simulink model "Gyro_Outage_Unit_Test"  (R2018b)
settings: Solver=VariableStepAuto  StartTime=0.0  StopTime=5600  FixedStep=fswParams.sample_time_s  RelTol=1e-8  AbsTol=1e-8
undefined symbols (not defined in the file or in its folder): B_eci_unit, Conversion_lib, DiscIntNeverNeededParam, e2sun_eci_unit, ECLIPSE, env_acc_mps2, Environment_lib, fswParams, gyro_body_radps, gyro_meas_valid, mag_body_T, mag_meas_valid, MEKF_Conversion_lib, MEKF_lib, photodiodes_A, q_body, r_eci_km, satelliteDynamics_lib, sc2sun_eci_unit, Sensors_Lib, simParams, solar_panel_power_W, sun_sensor_lib, sunsensor_2body_lib, sunsensor_body_deg, sunsensor_body_rad, sunsensor_valid, Triad, Triad_lib, v_eci_km, w_body_radps
libraries: aerolibutil x11, vrlib x10, sharedutil x8, simulink x5, dspmathops x4, sharedtransform x3, magnetometer_lib x3, gyroscope_lib x2, gravityGrad_Lib x1, atmoDrag_lib x1, magField_lib x1, solarPressure_lib x1
(part 2 of 3)

== system Gyro_Outage_Unit_Test/MEKF_lib1/Time Propagation (q,P) ==
  qe_plus : Inport
  P_chol_plus : Inport  Port=2
  Updated bias : Inport  Port=3
  omega_meas : Inport  Port=4
  Constant : Constant  Value=fswParams.estimation.dt
  Constant13 : Constant  Value=fswParams.estimation.Qchol  VectorParams1D=off
  Cross_Product_matrix : Subsystem
  Cross_product_matrix : Subsystem
  MATLAB Function : MATLAB Function  TreatAsAtomicUnit=on
  MATLAB Function10 : MATLAB Function  TreatAsAtomicUnit=on
  Matrix Multiply : Product  Multiplication=Matrix(*)
  Product : Product  Multiplication=Matrix(*)
  Psi : Subsystem
  Quaternion Normalize : sharedutil/Quaternion Normalize  aMode=aMode
      settings: SourceProductName=Aerospace Blockset  SourceProductBaseCode=AE
  Rate Transition : RateTransition  InitialCondition=fswParams.estimation.ic.Qchol_rt  OutPortSampleTime=fswParams.sample_time_s
  Sqrt : Sqrt  SaturateOnIntegerOverflow=on
  Subsystem : Subsystem
  Sum : Sum  Inputs=+-
  Transpose : Math  Operator=transpose  SaturateOnIntegerOverflow=on
  q_k_plus1 : Outport
  P_chol_plus_1 : Outport  Port=2
  Bias_Update : Outport  Port=3
  omega_est : Outport  Port=4
  wires:
  Quaternion Normalize/1 -> q_k_plus1/1
  omega_meas/1 -> Sum/1
  Product/1 -> Quaternion Normalize/1
  [del_t] -> MATLAB Function10/3(dt)
  qe_plus/1 -> Product/2
  [del_t] -> Psi/1(del_t)
  Sum/1 -> Cross_Product_matrix/1(omega_est), Matrix Multiply/2, omega_est/1, Psi/2(omega_vec), Transpose/1  "omega_estimate"
  Constant/1 -> [del_t]
  Matrix Multiply/1 -> Sqrt/1
  Transpose/1 -> Matrix Multiply/1
  Updated bias/1 -> Bias_Update/1, Sum/2
  Sqrt/1 -> MATLAB Function10/1(om_mag), Psi/3(omega_mag), Subsystem/4(omega_magnitude)  "omega_magnitude"
  Cross_Product_matrix/1(omega_x) -> MATLAB Function10/2(omega_x)
  [del_t] -> Subsystem/1(del_t)
  Psi/1(Psi1) -> Subsystem/3(Psi_vector), Cross_product_matrix/1(Psi_vec)  "Psi Vector"
  Cross_product_matrix/1(Psi_x) -> Subsystem/2(Psi_cross)
  Subsystem/1(OMEGA) -> Product/1
  Constant13/1 -> Rate Transition/1
  MATLAB Function10/1(Phi) -> MATLAB Function/2(Phi_discrete)  "State Transition Matrix"
  P_chol_plus/1 -> MATLAB Function/1("P_sq ")
  MATLAB Function/1(P_sq) -> P_chol_plus_1/1
  Rate Transition/1 -> MATLAB Function/3(Q_sq)

== system Gyro_Outage_Unit_Test/MEKF_lib1/Triad ==
  sc2sun_eci_unit : Inport
  B_eci_unit : Inport  Port=2
  sun_meas_rad_body : Inport  Port=3
  mag_meas_body_T : Inport  Port=4
  sunsensor_valid : Inport  Port=5
  magsensor_valid : Inport  Port=6
  Action Port : ActionPort
  Angle_between_vectors : Subsystem
  Bypass Triad : Subsystem  TreatAsAtomicUnit=on
  If : If  IfExpression=u1
  Logical Operator : Logic  Inputs=3  AllPortsSameDT=off  OutDataTypeStr=boolean
  Merge : Merge
  Quaternion Normalize : sharedutil/Quaternion Normalize  aMode=aMode
      settings: SourceProductName=Aerospace Blockset  SourceProductBaseCode=AE
  Triad_alg : Subsystem  TreatAsAtomicUnit=on
  Unit Delay : UnitDelay  InitialCondition=fswParams.estimation.ic.quat_est_init  SampleTime=fswParams.sample_time_s
  q_triad : Outport
  wires:
  Merge/1 -> Quaternion Normalize/1, [quat_old]
  Quaternion Normalize/1 -> q_triad/1
  If/1 -> Triad_alg/Action
  If/2 -> Bypass Triad/Action
  Triad_alg/1(quat_out 2) -> Merge/1
  Bypass Triad/1(quat_new) -> Merge/2
  Logical Operator/1 -> If/1
  sunsensor_valid/1 -> Logical Operator/1
  magsensor_valid/1 -> Logical Operator/2
  B_eci_unit/1 -> Triad_alg/3("mag_inertial ")
  [quat_old] -> Unit Delay/1
  Unit Delay/1 -> Bypass Triad/1(quat_old)
  sc2sun_eci_unit/1 -> Triad_alg/4(sun_inertial)
  sun_meas_rad_body/1 -> [sun_bod], Angle_between_vectors/1(sun_meas_rad_body)
  mag_meas_body_T/1 -> Angle_between_vectors/2(mag_meas_T_body), [meas_bod]
  Angle_between_vectors/1(Parallel_Protection) -> Logical Operator/3
  [sun_bod] -> Triad_alg/1(sun_body)
  [meas_bod] -> Triad_alg/2(mag_body)

== system Gyro_Outage_Unit_Test/MEKF_lib2/Angle_between_vectors ==
  sun_meas_rad_body : Inport
  mag_meas_T_body : Inport  Port=2
  Acos1 : Trigonometry  Commented=through  Operator=acos
  Divide : Product  Inputs=*/
  Dot Product : DotProduct  InputSameDT=on  OutDataTypeStr=Inherit: Inherit via internal rule
  Dot Product1 : DotProduct  InputSameDT=on  OutDataTypeStr=Inherit: Inherit via internal rule
  Dot Product2 : DotProduct  InputSameDT=on  OutDataTypeStr=Inherit: Inherit via internal rule
  Gain1 : Gain  Commented=through  Gain=180/pi
  MATLAB Function : MATLAB Function  TreatAsAtomicUnit=on
  Multiply : Product
  Multiply1 : Product
  Scope : Scope
  Sign : Signum
  Sqrt : Sqrt  SaturateOnIntegerOverflow=on
  Sqrt1 : Sqrt  SaturateOnIntegerOverflow=on
  Out1 : Outport
  wires:
  Dot Product1/1 -> Sqrt/1
  mag_meas_T_body/1 -> Dot Product2/2, Dot Product2/1, Dot Product/2
  sun_meas_rad_body/1 -> Dot Product1/1, Dot Product1/2, Dot Product/1
  Sqrt1/1 -> Multiply/2
  Sqrt/1 -> Multiply/1
  Dot Product/1 -> Divide/1
  Dot Product2/1 -> Sqrt1/1
  Multiply/1 -> Divide/2
  Acos1/1 -> Gain1/1
  Divide/1 -> Multiply1/1, Sign/1
  Multiply1/1 -> MATLAB Function/1(u)
  Sign/1 -> Multiply1/2
  MATLAB Function/1(y) -> Scope/1, Out1/1

== system Gyro_Outage_Unit_Test/MEKF_lib2/If Action Subsystem1 ==
  P (-) : Inport
  Bias (-) : Inport  Port=2
  q (-) : Inport  Port=3
  Action Port : ActionPort  ActionType=else
  q (+) : Outport
  P (+) : Outport  Port=2
  Bias (+) : Outport  Port=3
  wires:
  P (-)/1 -> P (+)/1
  Bias (-)/1 -> Bias (+)/1
  q (-)/1 -> q (+)/1

== system Gyro_Outage_Unit_Test/MEKF_lib2/If Action Subsystem2 ==
  In1 : Inport
  Action Port : ActionPort  ActionType=else
  Out1 : Outport
  wires:
  In1/1 -> Out1/1

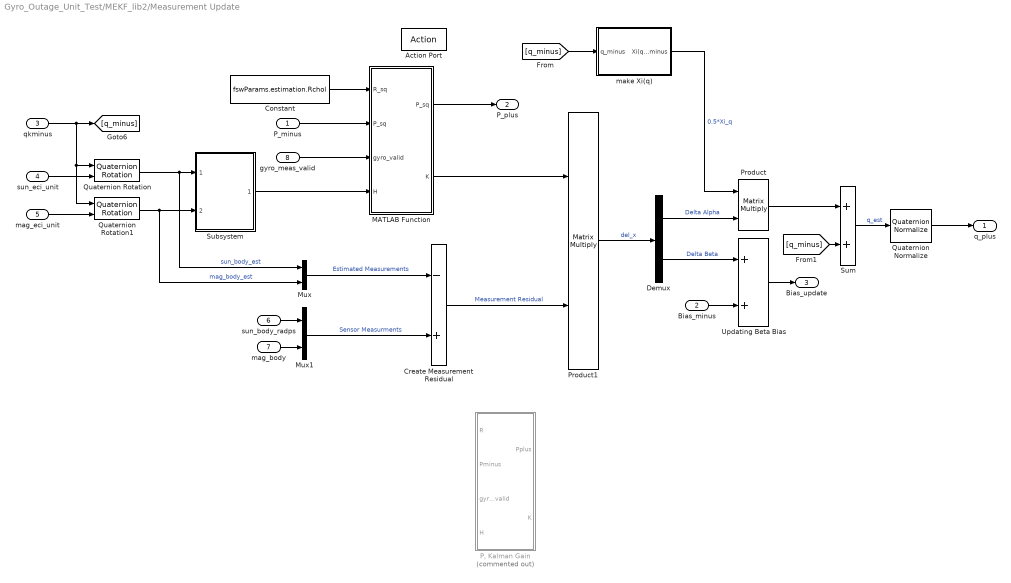
== system Gyro_Outage_Unit_Test/MEKF_lib2/Measurement Update ==
  P_minus : Inport
  Bias_minus : Inport  Port=2
  qkminus : Inport  Port=3
  sun_eci_unit : Inport  Port=4
  mag_eci_unit : Inport  Port=5
  sun_body_radps : Inport  Port=6
  mag_body : Inport  Port=7
  gyro_meas_valid : Inport  Port=8
  Action Port : ActionPort  ActionType=then
  Constant : Constant  Value=fswParams.estimation.Rchol  VectorParams1D=off
  Create Measurement Residual : Sum  Inputs=-+
  Demux : Demux  Outputs=2
  MATLAB Function : MATLAB Function  TreatAsAtomicUnit=on
  Mux : Mux  Inputs=2
  Mux1 : Mux  Inputs=2
  "P, Kalman Gain" : MATLAB Function  Commented=on  TreatAsAtomicUnit=on
  Product : Product  Inputs=**  Multiplication=Matrix(*)
  Product1 : Product  Multiplication=Matrix(*)
  Quaternion Normalize : sharedutil/Quaternion Normalize  aMode=aMode
      settings: SourceProductName=Aerospace Blockset  SourceProductBaseCode=AE
  Quaternion Rotation : aerolibutil/Quaternion Rotation
  Quaternion Rotation1 : aerolibutil/Quaternion Rotation
  Subsystem : Subsystem
  Sum : Sum
  "Updating Beta Bias " : Sum
  make Xi(q) : Subsystem
  q_plus : Outport
  P_plus : Outport  Port=2
  Bias_update : Outport  Port=3
  wires:
  MATLAB Function/2(K) -> Product1/1
  MATLAB Function/1(P_sq) -> P_plus/1
  Subsystem/1(H_matrix) -> MATLAB Function/4(H)
  gyro_meas_valid/1 -> MATLAB Function/3(gyro_valid)
  P_minus/1 -> MATLAB Function/2("P_sq ")
  Constant/1 -> MATLAB Function/1(R_sq)
  [q_minus] -> make Xi(q)/1(q_minus)
  qkminus/1 -> [q_minus], Quaternion Rotation/1, Quaternion Rotation1/1
  Quaternion Rotation/1 -> Mux/1, Subsystem/1(sun_body_hat)  "sun_body_est"
  Quaternion Rotation1/1 -> Mux/2, Subsystem/2(mag_body_hat)  "mag_body_est"
  mag_eci_unit/1 -> Quaternion Rotation1/2
  sun_eci_unit/1 -> Quaternion Rotation/2
  "Updating Beta Bias "/1 -> Bias_update/1
  sun_body_radps/1 -> Mux1/1
  mag_body/1 -> Mux1/2
  Create Measurement Residual/1 -> Product1/2  "Measurement Residual"
  make Xi(q)/1(Xi(q)_minus) -> Product/1  "0.5*Xi_q"
  Demux/1 -> Product/2  "Delta Alpha"
  Product1/1 -> Demux/1  "del_x"
  Product/1 -> Sum/1
  Sum/1 -> Quaternion Normalize/1  "q_est"
  Bias_minus/1 -> "Updating Beta Bias "/2
  Mux/1 -> Create Measurement Residual/1  "Estimated Measurements"
  Demux/2 -> "Updating Beta Bias "/1  "Delta Beta"
  Mux1/1 -> Create Measurement Residual/2  "Sensor Measurments"
  [q_minus] -> Sum/2
  Quaternion Normalize/1 -> q_plus/1

== system Gyro_Outage_Unit_Test/MEKF_lib2/Three_sigma ==
  P_plus : Inport
  Abs : Abs
  Demux : Demux  Outputs=2
  Extract Diagonal : S-Function  AncestorBlock=dspmtrx3/Extract Diagonal  FunctionName=sdspdiag2  Parameters=mode  SFunctionDeploymentMode=off  EnableBusSupport=off  mask(Extract Diagonal){}
      mask help: Extract the main diagonal of a full matrix.
      mask init:
      | mode = 2;
      | x = [.58 .87 NaN 0.12 0.45 0.45 0.12 0.12 NaN 0.525 0.525 0.475 0.475 0.525 0.525 0.565 0.525 ];
      | y = [ 0.8 0.2 NaN 0.2 0.2 0.8 0.8 0.2 NaN 0.435 0.475 0.475 0.525 0.525 0.565 0.5 0.435 ];
      mask Help: eval('blocksethelp');
      mask Display:
      | plot(x,y);
      | port_label('input',1,'A');
      | port_label('output',1,'D');
  Multiply : Gain  Gain=3*180/pi
  Terminator : Terminator
  3Sigma_deg : Outport
  wires:
  Demux/2 -> Terminator/1
  Demux/1 -> Abs/1
  Extract Diagonal/1 -> Demux/1
  Abs/1 -> Multiply/1
  P_plus/1 -> Extract Diagonal/1
  Multiply/1 -> 3Sigma_deg/1

== system Gyro_Outage_Unit_Test/MEKF_lib2/Time Propagation (q,P) ==
  qe_plus : Inport
  P_plus : Inport  Port=2
  Updated bias : Inport  Port=3
  omega_meas : Inport  Port=4
  Constant : Constant  Value=fswParams.estimation.dt
  Constant13 : Constant  Value=fswParams.estimation.Qchol  VectorParams1D=off
  Cross_Product_matrix : Subsystem
  Cross_product_matrix : Subsystem
  MATLAB Function : MATLAB Function  TreatAsAtomicUnit=on
  MATLAB Function1 : MATLAB Function  Commented=on  TreatAsAtomicUnit=on
  MATLAB Function10 : MATLAB Function  TreatAsAtomicUnit=on
  Matrix Multiply : Product  Multiplication=Matrix(*)
  Product : Product  Multiplication=Matrix(*)
  Psi : Subsystem
  Quaternion Normalize : sharedutil/Quaternion Normalize  aMode=aMode
      settings: SourceProductName=Aerospace Blockset  SourceProductBaseCode=AE
  Sqrt : Sqrt  SaturateOnIntegerOverflow=on
  Subsystem : Subsystem
  Sum : Sum  Inputs=+-
  Transpose : Math  Operator=transpose  SaturateOnIntegerOverflow=on
  P_k_plus1 : Outport
  q_k_plus1 : Outport  Port=2
  omega_est : Outport  Port=3
  Bias_Update : Outport  Port=4
  wires:
  MATLAB Function/1(P_sq) -> P_k_plus1/1
  P_plus/1 -> MATLAB Function/1("P_sq ")
  MATLAB Function10/1(Phi) -> MATLAB Function/2(Phi_discrete)  "State Transition Matrix"
  Constant13/1 -> MATLAB Function/3(Q_sq)
  Subsystem/1(OMEGA) -> Product/1
  Cross_product_matrix/1(Psi_x) -> Subsystem/2(Psi_cross)
  Psi/1(Psi1) -> Cross_product_matrix/1(Psi_vec), Subsystem/3(Psi_vector)  "Psi Vector"
  [del_t] -> Subsystem/1(del_t)
  Cross_Product_matrix/1(omega_x) -> MATLAB Function10/2(omega_x)
  Sqrt/1 -> Subsystem/4(omega_magnitude), Psi/3(omega_mag), MATLAB Function10/1(om_mag)  "omega_magnitude"
  Updated bias/1 -> Sum/2, Bias_Update/1
  Transpose/1 -> Matrix Multiply/1
  Matrix Multiply/1 -> Sqrt/1
  Constant/1 -> [del_t]
  Sum/1 -> Transpose/1, Psi/2(omega_vec), omega_est/1, Matrix Multiply/2, Cross_Product_matrix/1(omega_est)  "omega_estimate"
  [del_t] -> Psi/1(del_t)
  qe_plus/1 -> Product/2
  [del_t] -> MATLAB Function10/3(dt)
  Product/1 -> Quaternion Normalize/1
  omega_meas/1 -> Sum/1
  Quaternion Normalize/1 -> q_k_plus1/1

== system Gyro_Outage_Unit_Test/MEKF_lib2/Triad ==
  sc2sun_eci_unit : Inport
  B_eci_unit : Inport  Port=2
  sun_body_rad : Inport  Port=3
  mag_body_T : Inport  Port=4
  sunsensor_valid : Inport  Port=5
  magsensor_valid : Inport  Port=6
  Parallel_meas_check : Inport  Port=7
  Action Port : ActionPort  ActionType=then
  Bypass Triad : Subsystem  TreatAsAtomicUnit=on
  If : If  IfExpression=u1
  Logical Operator : Logic  Inputs=3  AllPortsSameDT=off  OutDataTypeStr=boolean
  Merge : Merge
  Quaternion Normalize : sharedutil/Quaternion Normalize  aMode=aMode
      settings: SourceProductName=Aerospace Blockset  SourceProductBaseCode=AE
  Triad_alg : Subsystem  TreatAsAtomicUnit=on
  Unit Delay : UnitDelay  InitialCondition=[0;0.707106781186547;0.707106781186547;0]  SampleTime=fswParams.sample_time_s
  q_triad : Outport
  wires:
  sc2sun_eci_unit/1 -> Triad_alg/4(sun_inertial)
  Unit Delay/1 -> Bypass Triad/1(quat_old)
  [quat_old] -> Unit Delay/1
  B_eci_unit/1 -> Triad_alg/3("mag_inertial ")
  sun_body_rad/1 -> Triad_alg/1(sun_body)
  mag_body_T/1 -> Triad_alg/2(mag_body)
  magsensor_valid/1 -> Logical Operator/2
  sunsensor_valid/1 -> Logical Operator/1
  Logical Operator/1 -> If/1
  Bypass Triad/1(quat_new) -> Merge/2
  Triad_alg/1(quat_out 2) -> Merge/1
  If/2 -> Bypass Triad/Action
  If/1 -> Triad_alg/Action
  Quaternion Normalize/1 -> q_triad/1
  Merge/1 -> [quat_old], Quaternion Normalize/1
  Parallel_meas_check/1 -> Logical Operator/3

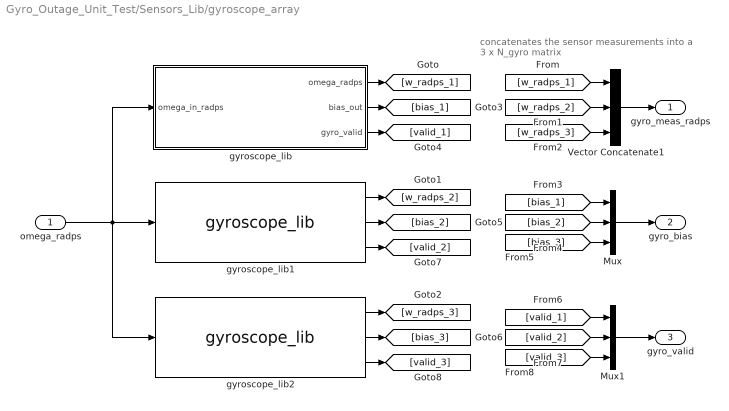
== system Gyro_Outage_Unit_Test/Sensors_Lib/gyroscope_array ==
  note: concatenates the sensor measurements
      | into a 3 x N_gyro matrix
  omega_radps : Inport
  Mux : Mux  Inputs=3
  Mux1 : Mux  Inputs=3
  Vector Concatenate1 : Concatenate  NumInputs=3  Mode=Multidimensional array  ConcatenateDimension=2
  gyroscope_lib : Subsystem  AncestorBlock=gyroscope_lib/gyroscope_lib  mask{id_s=1}
      mask prompts: id_s "Choose the sensor ID"
      mask TypeOptions id_s: 1 | 2 | 3
      mask DialogControl DescTextVar Prompt: SOCi gyroscope model. The spacecraft has three Bosch BMI055 gyroscopes.
  gyroscope_lib1 : gyroscope_lib/gyroscope_lib  id_s=2
  gyroscope_lib2 : gyroscope_lib/gyroscope_lib  id_s=3
  gyro_meas_radps : Outport
  gyro_bias : Outport  Port=2
  gyro_valid : Outport  Port=3
  wires:
  [valid_3] -> Mux1/3
  [valid_2] -> Mux1/2
  [valid_1] -> Mux1/1
  Mux1/1 -> gyro_valid/1
  [bias_3] -> Mux/3
  [bias_2] -> Mux/2
  [bias_1] -> Mux/1
  Mux/1 -> gyro_bias/1
  [w_radps_3] -> Vector Concatenate1/3
  [w_radps_2] -> Vector Concatenate1/2
  [w_radps_1] -> Vector Concatenate1/1
  Vector Concatenate1/1 -> gyro_meas_radps/1
  gyroscope_lib2/3 -> [valid_3]
  gyroscope_lib1/3 -> [valid_2]
  gyroscope_lib2/2 -> [bias_3]
  gyroscope_lib1/2 -> [bias_2]
  gyroscope_lib/3(gyro_valid) -> [valid_1]
  gyroscope_lib/2(bias_out) -> [bias_1]
  gyroscope_lib2/1 -> [w_radps_3]
  gyroscope_lib1/1 -> [w_radps_2]
  gyroscope_lib/1(omega_radps) -> [w_radps_1]
  omega_radps/1 -> gyroscope_lib1/1, gyroscope_lib/1(omega_in_radps), gyroscope_lib2/1

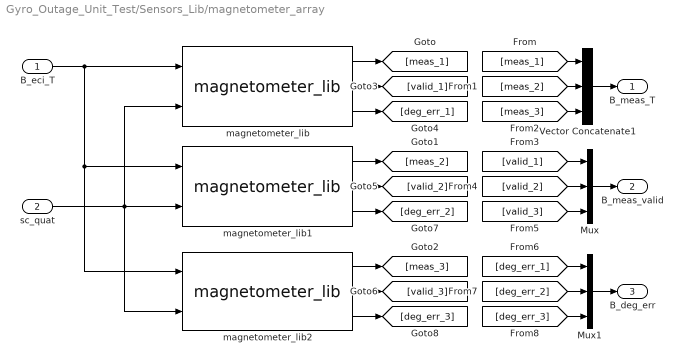
== system Gyro_Outage_Unit_Test/Sensors_Lib/magnetometer_array ==
  B_eci_T : Inport
  sc_quat : Inport  Port=2
  Mux : Mux  Inputs=3
  Mux1 : Mux  Inputs=3
  Vector Concatenate1 : Concatenate  NumInputs=3  Mode=Multidimensional array  ConcatenateDimension=2
  magnetometer_lib : magnetometer_lib/magnetometer_lib  id_s=1
  magnetometer_lib1 : magnetometer_lib/magnetometer_lib  id_s=2
  magnetometer_lib2 : magnetometer_lib/magnetometer_lib  id_s=1
  B_meas_T : Outport
  B_meas_valid : Outport  Port=2
  B_deg_err : Outport  Port=3
  wires:
  [deg_err_3] -> Mux1/3
  [deg_err_2] -> Mux1/2
  [deg_err_1] -> Mux1/1
  Mux1/1 -> B_deg_err/1
  [valid_3] -> Mux/3
  [valid_2] -> Mux/2
  [valid_1] -> Mux/1
  Mux/1 -> B_meas_valid/1
  [meas_3] -> Vector Concatenate1/3
  [meas_2] -> Vector Concatenate1/2
  [meas_1] -> Vector Concatenate1/1
  Vector Concatenate1/1 -> B_meas_T/1
  magnetometer_lib2/3 -> [deg_err_3]
  magnetometer_lib1/3 -> [deg_err_2]
  magnetometer_lib2/2 -> [valid_3]
  magnetometer_lib1/2 -> [valid_2]
  magnetometer_lib/3 -> [deg_err_1]
  magnetometer_lib/2 -> [valid_1]
  magnetometer_lib2/1 -> [meas_3]
  magnetometer_lib1/1 -> [meas_2]
  magnetometer_lib/1 -> [meas_1]
  B_eci_T/1 -> magnetometer_lib1/1, magnetometer_lib2/1, magnetometer_lib/1
  sc_quat/1 -> magnetometer_lib1/2, magnetometer_lib2/2, magnetometer_lib/2

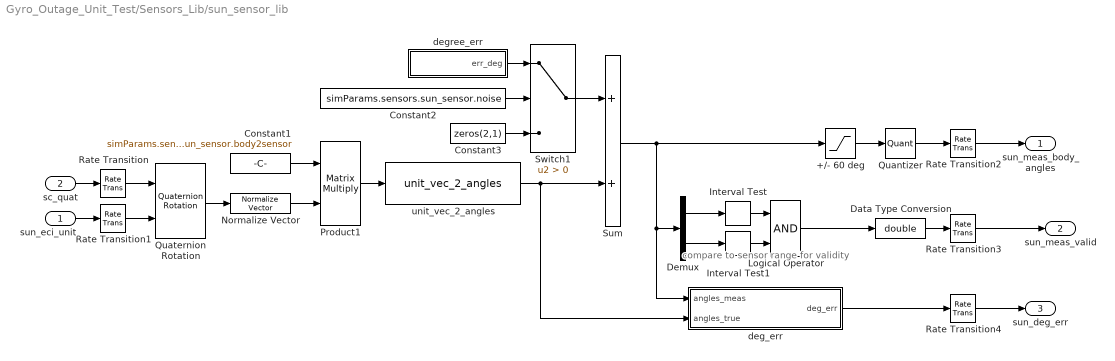
== system Gyro_Outage_Unit_Test/Sensors_Lib/sun_sensor_lib  ==
  note: compare to sensor range for validity
  sun_eci_unit : Inport
  sc_quat : Inport  Port=2
  +/- 60 deg : Saturate  UpperLimit=simParams.sensors.sun_sensor.range_deg  LowerLimit=-simParams.sensors.sun_sensor.range_deg
  Constant1 : Constant  Value=simParams.sensors.sun_sensor.body2sensor
  Constant2 : Constant  Value=simParams.sensors.sun_sensor.noise
  Constant3 : Constant  Value=zeros(2,1)
  Data Type Conversion : DataTypeConversion  OutDataTypeStr=double
  Demux : Demux  Outputs=2
  Interval Test : simulink/Logic and Bit Operations/Interval Test  IntervalClosedRight=on  uplimit=simParams.sensors.sun_sensor.range_deg  IntervalClosedLeft=on  lowlimit=-simParams.sensors.sun_sensor.range_deg  OutDataTypeStr=boolean
  Interval Test1 : simulink/Logic and Bit Operations/Interval Test  IntervalClosedRight=on  uplimit=simParams.sensors.sun_sensor.range_deg  IntervalClosedLeft=on  lowlimit=-simParams.sensors.sun_sensor.range_deg  OutDataTypeStr=boolean
  Logical Operator : Logic  AllPortsSameDT=off  OutDataTypeStr=boolean
  Normalize Vector : vrlib/Utilities/Normalize Vector  maxzero=0
      settings: SourceProductName=Simulink 3D Animation  SourceProductBaseCode=VR
  Product1 : Product  Multiplication=Matrix(*)  RndMeth=Zero
  Quantizer : Quantizer  QuantizationInterval=simParams.sensors.sun_sensor.resolution
  Quaternion Rotation : aerolibutil/Quaternion Rotation
  Rate Transition : RateTransition  InitialCondition=simParams.initialConditions.q0  OutPortSampleTime=simParams.sensors.sun_sensor.sample_time_s
  Rate Transition1 : RateTransition  OutPortSampleTime=simParams.sensors.sun_sensor.sample_time_s
  Rate Transition2 : RateTransition
  Rate Transition3 : RateTransition
  Rate Transition4 : RateTransition
  Sum : Sum
  Switch1 : Switch  Criteria=u2 > Threshold
  deg_err : Subsystem
  degree_err : Subsystem
  unit_vec_2_angles : ss_vec_2_angles/unit_vec_2_angles  SystemSampleTime=-1
  sun_meas_body_angles : Outport
  sun_meas_valid : Outport  Port=2
  sun_deg_err : Outport  Port=3
  wires:
  Rate Transition4/1 -> sun_deg_err/1
  Rate Transition2/1 -> sun_meas_body_angles/1
  Rate Transition1/1 -> Quaternion Rotation/2
  Rate Transition/1 -> Quaternion Rotation/1
  Data Type Conversion/1 -> Rate Transition3/1
  Demux/2 -> Interval Test1/1
  Sum/1 -> Demux/1, deg_err/1(angles_meas), +/- 60 deg/1
  unit_vec_2_angles/1 -> deg_err/2(angles_true), Sum/2
  Product1/1 -> unit_vec_2_angles/1
  Constant1/1 -> Product1/1
  +/- 60 deg/1 -> Quantizer/1
  Logical Operator/1 -> Data Type Conversion/1
  Interval Test1/1 -> Logical Operator/2
  Interval Test/1 -> Logical Operator/1
  Demux/1 -> Interval Test/1
  Normalize Vector/1 -> Product1/2
  Quantizer/1 -> Rate Transition2/1
  Quaternion Rotation/1 -> Normalize Vector/1
  degree_err/1("err_deg ") -> Switch1/1
  deg_err/1(deg_err) -> Rate Transition4/1
  sun_eci_unit/1 -> Rate Transition1/1
  Switch1/1 -> Sum/1
  Constant3/1 -> Switch1/3
  Constant2/1 -> Switch1/2
  sc_quat/1 -> Rate Transition/1
  Rate Transition3/1 -> sun_meas_valid/1

== system Gyro_Outage_Unit_Test/satelliteDynamics_lib/RigidBodyDynamics ==
  external_torque : Inport
  RW_torque : Inport  Port=2
  Integrator : Integrator  InitialCondition=[0;0;0]
  dynamics : Subsystem
  wint : Integrator  InitialCondition=[0.01;0.005;0]  AbsoluteTolerance=1e-10
  body_rates : Outport
  wires:
  external_torque/1 -> dynamics/1(external_torque_Nm)
  Integrator/1 -> dynamics/3(rw_momentum_Nms)
  RW_torque/1 -> Integrator/1, dynamics/2(rw_torque_Nm)
  dynamics/1(omega_dot) -> wint/1
  wint/1 -> dynamics/4(omega_radps), body_rates/1

== system Gyro_Outage_Unit_Test/satelliteDynamics_lib/quat_propagation ==
  body_rates : Inport
  Gain1 : Gain  Gain=1/2
  Integrator : Integrator  InitialCondition=[0;0.707106781186547;0.707106781186547;0]
  MATLAB Function : MATLAB Function  TreatAsAtomicUnit=on
  Product : Product  Multiplication=Matrix(*)  RndMeth=Zero
  Quaternion Normalize : sharedutil/Quaternion Normalize  aMode=aMode
      settings: SourceProductName=Aerospace Blockset  SourceProductBaseCode=AE
  Scope : Scope
  quat : Outport
  wires:
  Quaternion Normalize/1 -> Scope/1, Product/2, quat/1
  Gain1/1 -> Product/1
  body_rates/1 -> MATLAB Function/1(w)
  MATLAB Function/1(Omega) -> Gain1/1
  Product/1 -> Integrator/1
  Integrator/1 -> Quaternion Normalize/1

== system Gyro_Outage_Unit_Test/Conversion_lib/sunsensor_body_rad1/Create_Sz ==
  alpha : Inport
  beta : Inport  Port=2
  Constant : Constant
  Math Function : Math  Operator=square  SaturateOnIntegerOverflow=on
  Math Function1 : Math  Operator=square  SaturateOnIntegerOverflow=on
  Math Function2 : Math  Operator=reciprocal  SaturateOnIntegerOverflow=on
  Sqrt : Sqrt  SaturateOnIntegerOverflow=on
  Sum : Sum  Inputs=|+++
  Tan : Trigonometry  Operator=tan
  Tan1 : Trigonometry  Operator=tan
  Out1 : Outport
  wires:
  Constant/1 -> Sum/1
  Sum/1 -> Math Function2/1
  Tan/1 -> Math Function/1
  Math Function/1 -> Sum/2
  Math Function2/1 -> Sqrt/1
  Tan1/1 -> Math Function1/1
  alpha/1 -> Tan/1
  beta/1 -> Tan1/1
  Math Function1/1 -> Sum/3
  Sqrt/1 -> Out1/1

== system Gyro_Outage_Unit_Test/MEKF_lib1/MEKF or Propagation/Angle_between_vectors ==
  sun_meas_rad_body : Inport
  mag_meas_T_body : Inport  Port=2
  Divide : Product  Inputs=*/
  Dot Product : DotProduct  InputSameDT=on  OutDataTypeStr=Inherit: Inherit via internal rule
  Dot Product1 : DotProduct  InputSameDT=on  OutDataTypeStr=Inherit: Inherit via internal rule
  Dot Product2 : DotProduct  InputSameDT=on  OutDataTypeStr=Inherit: Inherit via internal rule
  MATLAB Function : MATLAB Function  TreatAsAtomicUnit=on
  Multiply : Product
  Sqrt : Sqrt  SaturateOnIntegerOverflow=on
  Sqrt1 : Sqrt  SaturateOnIntegerOverflow=on
  Parallel_Protection : Outport
  wires:
  Dot Product1/1 -> Sqrt/1
  mag_meas_T_body/1 -> Dot Product2/2, Dot Product2/1, Dot Product/2
  sun_meas_rad_body/1 -> Dot Product1/1, Dot Product1/2, Dot Product/1
  Sqrt1/1 -> Multiply/2
  Sqrt/1 -> Multiply/1
  Dot Product/1 -> Divide/1
  Dot Product2/1 -> Sqrt1/1
  Multiply/1 -> Divide/2
  Divide/1 -> MATLAB Function/1(u)
  MATLAB Function/1(y) -> Parallel_Protection/1

== system Gyro_Outage_Unit_Test/MEKF_lib1/Measurement Update/Subsystem ==
  sun_body_hat : Inport
  mag_body_hat : Inport  Port=2
  Constant1 : Constant  Value=zeros(3,3)  VectorParams1D=off
  Constant2 : Constant  Value=zeros(3,3)  VectorParams1D=off
  Cross_product_matrix2 : Subsystem
  Cross_product_matrix3 : Subsystem
  Horizontal Matrix Concatenate : Concatenate  Mode=Multidimensional array
  Horizontal Matrix Concatenate1 : Concatenate  Mode=Multidimensional array
  Vertical Matrix Concatenate : Concatenate  Mode=Multidimensional array  ConcatenateDimension=2
  H_matrix : Outport
  wires:
  Vertical Matrix Concatenate/1 -> H_matrix/1
  mag_body_hat/1 -> Cross_product_matrix3/1(mag_body_hat)
  Cross_product_matrix2/1(sun_body_x) -> Horizontal Matrix Concatenate/1
  sun_body_hat/1 -> Cross_product_matrix2/1(sun_body_hat)
  Horizontal Matrix Concatenate1/1 -> Vertical Matrix Concatenate/2
  Horizontal Matrix Concatenate/1 -> Vertical Matrix Concatenate/1
  Cross_product_matrix3/1(mag_body_x) -> Horizontal Matrix Concatenate/2
  Constant2/1 -> Horizontal Matrix Concatenate1/1
  Constant1/1 -> Horizontal Matrix Concatenate1/2

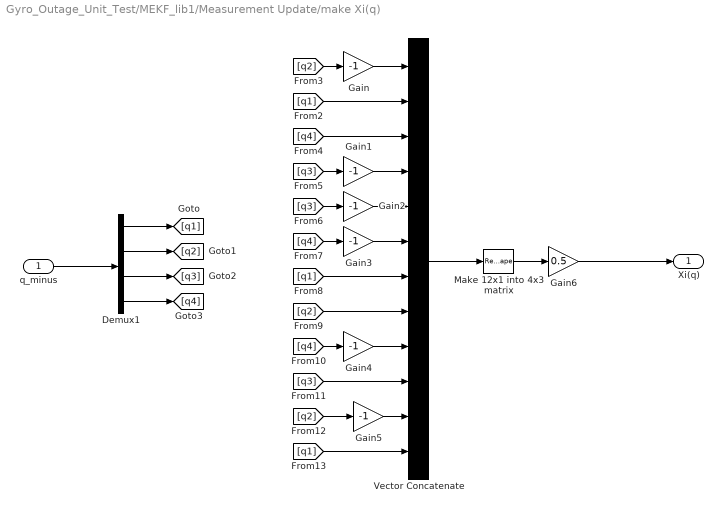
== system Gyro_Outage_Unit_Test/MEKF_lib1/Measurement Update/make Xi(q) ==
  q_minus : Inport
  Demux1 : Demux
  Gain{,1..5} (6 alike) : Gain  Gain=-1
  Gain6 : Gain  Gain=0.5
  Make 12x1 into 4x3 matrix : Reshape  OutputDimensionality=Customize  OutputDimensions=[4,3]
  Vector Concatenate : Concatenate  NumInputs=12
  Xi(q) : Outport
  wires:
  Gain6/1 -> Xi(q)/1
  q_minus/1 -> Demux1/1
  Demux1/4 -> [q4]
  [q1] -> Vector Concatenate/7
  Gain5/1 -> Vector Concatenate/11
  [q4] -> Gain4/1
  [q2] -> Gain5/1
  Gain/1 -> Vector Concatenate/1
  [q1] -> Vector Concatenate/12
  [q4] -> Vector Concatenate/3
  Demux1/3 -> [q3]
  Gain4/1 -> Vector Concatenate/9
  Demux1/1 -> [q1]
  [q2] -> Vector Concatenate/8
  Demux1/2 -> [q2]
  Gain1/1 -> Vector Concatenate/4
  Gain2/1 -> Vector Concatenate/5
  [q3] -> Vector Concatenate/10
  [q2] -> Gain/1
  [q4] -> Gain3/1
  [q3] -> Gain1/1
  Make 12x1 into 4x3 matrix/1 -> Gain6/1
  [q1] -> Vector Concatenate/2
  Gain3/1 -> Vector Concatenate/6
  [q3] -> Gain2/1
  Vector Concatenate/1 -> Make 12x1 into 4x3 matrix/1

== system Gyro_Outage_Unit_Test/MEKF_lib1/Subsystem/If Action Subsystem2 ==
  In1 : Inport
  Action Port : ActionPort  ActionType=else
  Out1 : Outport
  wires:
  In1/1 -> Out1/1

== system Gyro_Outage_Unit_Test/MEKF_lib1/Time Propagation (q,P)/Cross_Product_matrix ==
  omega_est : Inport
  Constant1 : Constant  Value=0
  Constant2 : Constant  Value=0
  Constant3 : Constant  Value=0
  Demux1 : Demux  Outputs=3
  Gain : Gain  Gain=-1
  Gain1 : Gain  Gain=-1
  Gain3 : Gain  Gain=-1
  Makes Cross Product Matrix : Reshape  OutputDimensionality=Customize  OutputDimensions=[3,3]
  Vector Concatenate : Concatenate  NumInputs=9
  omega_x : Outport
  wires:
  Vector Concatenate/1 -> Makes Cross Product Matrix/1
  Demux1/2 -> [v2]
  Demux1/1 -> [v1]
  Demux1/3 -> [v3]
  [v2] -> Vector Concatenate/7
  Constant3/1 -> Vector Concatenate/9
  [v1] -> Vector Concatenate/6
  omega_est/1 -> Demux1/1
  [v1] -> Gain1/1
  [v3] -> Vector Concatenate/2
  Constant1/1 -> Vector Concatenate/1
  Constant2/1 -> Vector Concatenate/5
  Makes Cross Product Matrix/1 -> omega_x/1
  [v3] -> Gain3/1
  [v2] -> Gain/1
  Gain/1 -> Vector Concatenate/3
  Gain3/1 -> Vector Concatenate/4
  Gain1/1 -> Vector Concatenate/8

== system Gyro_Outage_Unit_Test/MEKF_lib1/Time Propagation (q,P)/Cross_product_matrix ==
  Psi_vec : Inport
  Constant1 : Constant  Value=0
  Constant2 : Constant  Value=0
  Constant3 : Constant  Value=0
  Demux1 : Demux  Outputs=3
  Gain : Gain  Gain=-1
  Gain1 : Gain  Gain=-1
  Gain3 : Gain  Gain=-1
  Makes Cross Product Matrix : Reshape  OutputDimensionality=Customize  OutputDimensions=[3,3]
  Vector Concatenate : Concatenate  NumInputs=9
  Psi_x : Outport
  wires:
  Constant3/1 -> Vector Concatenate/9
  [v3] -> Gain3/1
  [v2] -> Gain/1
  Demux1/3 -> [v3]
  Makes Cross Product Matrix/1 -> Psi_x/1
  Psi_vec/1 -> Demux1/1
  Gain/1 -> Vector Concatenate/3
  Gain1/1 -> Vector Concatenate/8
  Vector Concatenate/1 -> Makes Cross Product Matrix/1
  Demux1/2 -> [v2]
  [v3] -> Vector Concatenate/2
  Constant1/1 -> Vector Concatenate/1
  [v2] -> Vector Concatenate/7
  [v1] -> Vector Concatenate/6
  Constant2/1 -> Vector Concatenate/5
  Gain3/1 -> Vector Concatenate/4
  [v1] -> Gain1/1
  Demux1/1 -> [v1]

== system Gyro_Outage_Unit_Test/MEKF_lib1/Time Propagation (q,P)/Psi ==
  del_t : Inport
  omega_vec : Inport  Port=2
  omega_mag : Inport  Port=3
  If : If  IfExpression=u1<1e-10
  If Action Subsystem : Subsystem  TreatAsAtomicUnit=on
  If Action Subsystem1 : Subsystem  TreatAsAtomicUnit=on
  Merge : Merge
  Psi1 : Outport
  wires:
  If/2 -> If Action Subsystem/Action
  If Action Subsystem/1(Psi) -> Merge/2
  If/1 -> If Action Subsystem1/Action
  If Action Subsystem1/1(Psi_zero) -> Merge/1
  Merge/1 -> Psi1/1
  omega_vec/1 -> If Action Subsystem/2(omega_vec)
  del_t/1 -> If Action Subsystem/1(del_t)
  omega_mag/1 -> If Action Subsystem/3(omega_mag), If/1

== system Gyro_Outage_Unit_Test/MEKF_lib1/Time Propagation (q,P)/Subsystem ==
  del_t : Inport
  Psi_cross : Inport  Port=2
  Psi_vector : Inport  Port=3
  omega_magnitude : Inport  Port=4
  Add1 : Sum  Inputs=+-
  Constant : Constant  Value=0.5
  Cos : Trigonometry  Operator=cos
  Gain : Gain  Gain=-1
  Identity Matrix : S-Function  FunctionName=sdspeye  Parameters=Inherit,N,Ts,isCustomFloat,fxpIsSigned,dTypeID,fxpWordLength,fxpFracLength,1  SFunctionDeploymentMode=off  EnableBusSupport=off  mask(Identity Matrix){Inherit=off, N=3, Ts=1, additionalParams=off, allowOverrides=on, dataType=double, isSigned=on, wordLen=16, udDataType=sfix(16), fracBitsMode=Best precision, numFracBits=15, OutDataTypeStr=double, LastOutDataTypeStr=double}
      mask prompts: Inherit "Inherit output port attributes from input port"; N "Matrix size:"; Ts "Sample time:"; additionalParams "------- Show additional parameters --------"; allowOverrides "Allow overrides by DSP Fixed-Point Attributes blocks"; dataType "Output data type:"; isSigned "Signed"; wordLen "Word length:"; udDataType "User-defined data type (e.g. sfix(16), float('single')):"; fracBitsMode "Set fraction length in output to:"; numFracBits "Fraction length:"; OutDataTypeStr "Output data type:"; LastOutDataTypeStr "Last output data type:"
      mask help: Output an identity matrix. If the matrix size entered is a scalar, then the output will be a square (symmetric) identity matrix with the number of rows and columns both equal to the specified value. If the matrix size entered is a two-element vector [M N], then the output will be an asymmetric matrix with the number of rows equal to M, the number of columns equal to N, ones down the diagonal, and zeros elsewhere. This matches the syntax of the MATLAB function eye(N) and eye(M,N), respectively.
      mask init:
      | isCustomFloat =  0; % nice default
      | fxpIsSigned   =  1; % nice default
      | fxpWordLength =  8; % nice default
      | fxpFracLength =  0; % nice default
      | if Inherit
      |     dTypeID   = -3; % SAME_AS_INPUT
      | else
      |     dtRows            = dspblkGetDiscreteImpulseDTRowInfo();
      |     [dtInfo, dTypeID] = dspblkUDTMapperOutDType(gcbh, dtRows{1}, 'dataType', 1.0);
      |     isCustomFloat     = dtInfo.DataTypeIsCustomFloat;
      |     if ~isCustomFloat
      |         fxpIsSigned   = dtInfo.DataTypeIsSigned;
      |         fxpWordLength = dtInfo.DataTypeWordLength;
      |         fxpFracLength = dtInfo.DataTypeFracOrMantBits;
      |     end
      | end
      mask Help: eval('blocksethelp');
      mask Callback Inherit: dspblkeye
      mask TypeOptions dataType: double | single | int8 | uint8 | int16 | uint16 | int32 | uint32 | boolean | Fixed-point | User-defined | Inherit via back propagation
      mask TypeOptions fracBitsMode: Best precision | User-defined
      mask Display:
      | if Inherit
      |     disp('eye( )');
      | else
      |     disp(['eye(' , num2str(get_param(gcbh, 'N')), ')']);
      | end
  Matrix Concatenate : Concatenate  Mode=Multidimensional array  ConcatenateDimension=2
  Matrix Concatenate1 : Concatenate  Mode=Multidimensional array  ConcatenateDimension=2
  Matrix Concatenate2 : Concatenate  Mode=Multidimensional array
  Matrix Multiply2 : Product
  Multiply : Product  Inputs=3
  Transpose2 : Math  Operator=transpose  SaturateOnIntegerOverflow=on
  OMEGA : Outport
  wires:
  Matrix Concatenate2/1 -> OMEGA/1
  Multiply/1 -> Cos/1
  Matrix Multiply2/1 -> Add1/1
  Add1/1 -> Matrix Concatenate1/2
  Matrix Concatenate1/1 -> Matrix Concatenate2/2
  Matrix Concatenate/1 -> Matrix Concatenate2/1
  Psi_vector/1 -> Gain/1, Matrix Concatenate1/1
  Cos/1 -> Matrix Concatenate/1, Matrix Multiply2/1
  Transpose2/1 -> Matrix Concatenate/2
  Psi_cross/1 -> Add1/2
  Identity Matrix/1 -> Matrix Multiply2/2
  del_t/1 -> Multiply/1
  omega_magnitude/1 -> Multiply/3
  Constant/1 -> Multiply/2
  Gain/1 -> Transpose2/1

== system Gyro_Outage_Unit_Test/MEKF_lib1/Triad/Angle_between_vectors ==
  sun_meas_rad_body : Inport
  mag_meas_T_body : Inport  Port=2
  Divide : Product  Inputs=*/
  Dot Product : DotProduct  InputSameDT=on  OutDataTypeStr=Inherit: Inherit via internal rule
  Dot Product1 : DotProduct  InputSameDT=on  OutDataTypeStr=Inherit: Inherit via internal rule
  Dot Product2 : DotProduct  InputSameDT=on  OutDataTypeStr=Inherit: Inherit via internal rule
  MATLAB Function : MATLAB Function  TreatAsAtomicUnit=on
  Multiply : Product
  Sqrt : Sqrt  SaturateOnIntegerOverflow=on
  Sqrt1 : Sqrt  SaturateOnIntegerOverflow=on
  Parallel_Protection : Outport
  wires:
  Dot Product1/1 -> Sqrt/1
  mag_meas_T_body/1 -> Dot Product2/2, Dot Product2/1, Dot Product/2
  sun_meas_rad_body/1 -> Dot Product1/1, Dot Product1/2, Dot Product/1
  Sqrt1/1 -> Multiply/2
  Sqrt/1 -> Multiply/1
  Dot Product/1 -> Divide/1
  Dot Product2/1 -> Sqrt1/1
  Multiply/1 -> Divide/2
  Divide/1 -> MATLAB Function/1(u)
  MATLAB Function/1(y) -> Parallel_Protection/1

== system Gyro_Outage_Unit_Test/MEKF_lib1/Triad/Bypass Triad ==
  quat_old : Inport
  Action Port : ActionPort
  quat_new : Outport
  wires:
  quat_old/1 -> quat_new/1

== system Gyro_Outage_Unit_Test/MEKF_lib1/Triad/Triad_alg ==
  sun_body : Inport
  mag_body : Inport  Port=2
  "mag_inertial " : Inport  Port=3
  sun_inertial : Inport  Port=4
  Action Port : ActionPort
  Cross Product{4..7} (4 alike) : vrlib/Utilities/Cross Product
      settings: SourceProductBaseCode=VR
  Direction Cosine Matrix to Quaternions2 : sharedtransform/Direction Cosine Matrix  to Quaternions  aMode=0  action=None  tolerance=eps(2)
      settings: SourceProductName=Aerospace Blockset  SourceProductBaseCode=AE
  Math Function1 : Math  Operator=transpose  SaturateOnIntegerOverflow=on
  Matrix Concatenate2 : Concatenate  NumInputs=3  Mode=Multidimensional array  ConcatenateDimension=2
  Matrix Concatenate3 : Concatenate  NumInputs=3  Mode=Multidimensional array  ConcatenateDimension=2
  Matrix Multiply1 : Product  Multiplication=Matrix(*)
  Multiply : Product
  Normalization6 : dspmathops/Normalization  NormType=2-norm  Bias=1e-10  NormOver=Each column  Dimension=1  roundingMode=Floor  overflowMode=off  accumDataTypeStr=Inherit: Same as product output  accumLastDataTypeStr=Inherit: Same as product output  outputDataTypeStr=Inherit: Same as product output  outputMin=[]  outputMax=[]  outputLastDataTypeStr=Inherit: Same as product output
      settings: SourceProductName=DSP System Toolbox
  Normalization7 : dspmathops/Normalization  NormType=2-norm  Bias=1e-10  NormOver=Each column  Dimension=1  roundingMode=Floor  overflowMode=off  accumDataTypeStr=Inherit: Same as product output  accumLastDataTypeStr=Inherit: Same as product output  outputDataTypeStr=Inherit: Same as product output  outputMin=[]  outputMax=[]  outputLastDataTypeStr=Inherit: Same as product output
      settings: SourceProductName=DSP System Toolbox
  Selector : Selector  InputPortWidth=4  IndexOptions=Index vector (dialog)  Indices=[1]  OutputSizes=1
  Sign : Signum
  quat_out 2 : Outport
  wires:
  sun_body/1 -> Matrix Concatenate2/1, Cross Product5/1, Cross Product4/1
  mag_body/1 -> Cross Product4/2
  Cross Product4/1 -> Normalization6/1  "S x M"
  Normalization6/1 -> Matrix Concatenate2/2, Cross Product5/2  "M"
  Cross Product5/1 -> Matrix Concatenate2/3  "S x M"
  sun_inertial/1 -> Cross Product6/1, Matrix Concatenate3/1, Cross Product7/1
  Cross Product7/1 -> Matrix Concatenate3/3  "S x M"
  Normalization7/1 -> Matrix Concatenate3/2, Cross Product7/2  "M"
  Cross Product6/1 -> Normalization7/1  "S x M"
  "mag_inertial "/1 -> Cross Product6/2
  Matrix Concatenate3/1 -> Math Function1/1
  Matrix Multiply1/1 -> Direction Cosine Matrix to Quaternions2/1
  Matrix Concatenate2/1 -> [dcm_body]
  Math Function1/1 -> [dcm_Inert]
  [dcm_body] -> Matrix Multiply1/1
  [dcm_Inert] -> Matrix Multiply1/2
  Direction Cosine Matrix to Quaternions2/1 -> Multiply/2, Selector/1
  Sign/1 -> Multiply/1
  Selector/1 -> Sign/1
  Multiply/1 -> quat_out 2/1

== system Gyro_Outage_Unit_Test/MEKF_lib2/Measurement Update/Subsystem ==
  sun_body_hat : Inport
  mag_body_hat : Inport  Port=2
  Constant1 : Constant  Value=zeros(3,3)  VectorParams1D=off
  Constant2 : Constant  Value=zeros(3,3)  VectorParams1D=off
  Cross_product_matrix2 : Subsystem  AncestorBlock=MEKF_lib/MEKF_lib/Measurement Update/Cross_product_matrix
  Cross_product_matrix3 : Subsystem  AncestorBlock=MEKF_lib/MEKF_lib/Measurement Update/Cross_product_matrix1
  Horizontal Matrix Concatenate : Concatenate  Mode=Multidimensional array
  Horizontal Matrix Concatenate1 : Concatenate  Mode=Multidimensional array
  Vertical Matrix Concatenate : Concatenate  Mode=Multidimensional array  ConcatenateDimension=2
  H_matrix : Outport
  wires:
  Constant1/1 -> Horizontal Matrix Concatenate1/2
  Constant2/1 -> Horizontal Matrix Concatenate1/1
  Cross_product_matrix3/1(mag_body_x) -> Horizontal Matrix Concatenate/2
  Horizontal Matrix Concatenate/1 -> Vertical Matrix Concatenate/1
  Horizontal Matrix Concatenate1/1 -> Vertical Matrix Concatenate/2
  sun_body_hat/1 -> Cross_product_matrix2/1(sun_body_hat)
  Cross_product_matrix2/1(sun_body_x) -> Horizontal Matrix Concatenate/1
  mag_body_hat/1 -> Cross_product_matrix3/1(mag_body_hat)
  Vertical Matrix Concatenate/1 -> H_matrix/1

== system Gyro_Outage_Unit_Test/MEKF_lib2/Measurement Update/make Xi(q) ==
  q_minus : Inport
  Demux1 : Demux
  Gain{,1..5} (6 alike) : Gain  Gain=-1
  Gain6 : Gain  Gain=0.5
  Make 12x1 into 4x3 matrix : Reshape  OutputDimensionality=Customize  OutputDimensions=[4,3]
  Vector Concatenate : Concatenate  NumInputs=12
  Xi(q)_minus : Outport
  wires:
  Vector Concatenate/1 -> Make 12x1 into 4x3 matrix/1
  [q3] -> Gain2/1
  Gain3/1 -> Vector Concatenate/6
  [q1] -> Vector Concatenate/2
  Make 12x1 into 4x3 matrix/1 -> Gain6/1
  [q3] -> Gain1/1
  [q4] -> Gain3/1
  [q2] -> Gain/1
  [q3] -> Vector Concatenate/10
  Gain2/1 -> Vector Concatenate/5
  Gain1/1 -> Vector Concatenate/4
  Demux1/2 -> [q2]
  [q2] -> Vector Concatenate/8
  Demux1/1 -> [q1]
  Gain4/1 -> Vector Concatenate/9
  Demux1/3 -> [q3]
  [q4] -> Vector Concatenate/3
  [q1] -> Vector Concatenate/12
  Gain/1 -> Vector Concatenate/1
  [q2] -> Gain5/1
  [q4] -> Gain4/1
  Gain5/1 -> Vector Concatenate/11
  [q1] -> Vector Concatenate/7
  Demux1/4 -> [q4]
  q_minus/1 -> Demux1/1
  Gain6/1 -> Xi(q)_minus/1

== system Gyro_Outage_Unit_Test/MEKF_lib2/Time Propagation (q,P)/Cross_Product_matrix ==
  omega_est : Inport
  Constant1 : Constant  Value=0
  Constant2 : Constant  Value=0
  Constant3 : Constant  Value=0
  Demux1 : Demux  Outputs=3
  Gain : Gain  Gain=-1
  Gain1 : Gain  Gain=-1
  Gain3 : Gain  Gain=-1
  Makes Cross Product Matrix : Reshape  OutputDimensionality=Customize  OutputDimensions=[3,3]
  Vector Concatenate : Concatenate  NumInputs=9
  omega_x : Outport
  wires:
  Gain1/1 -> Vector Concatenate/8
  Gain3/1 -> Vector Concatenate/4
  Gain/1 -> Vector Concatenate/3
  [v2] -> Gain/1
  [v3] -> Gain3/1
  Makes Cross Product Matrix/1 -> omega_x/1
  Constant2/1 -> Vector Concatenate/5
  Constant1/1 -> Vector Concatenate/1
  [v3] -> Vector Concatenate/2
  [v1] -> Gain1/1
  omega_est/1 -> Demux1/1
  [v1] -> Vector Concatenate/6
  Constant3/1 -> Vector Concatenate/9
  [v2] -> Vector Concatenate/7
  Demux1/3 -> [v3]
  Demux1/1 -> [v1]
  Demux1/2 -> [v2]
  Vector Concatenate/1 -> Makes Cross Product Matrix/1

== system Gyro_Outage_Unit_Test/MEKF_lib2/Time Propagation (q,P)/Cross_product_matrix ==
  Psi_vec : Inport
  Constant1 : Constant  Value=0
  Constant2 : Constant  Value=0
  Constant3 : Constant  Value=0
  Demux1 : Demux  Outputs=3
  Gain : Gain  Gain=-1
  Gain1 : Gain  Gain=-1
  Gain3 : Gain  Gain=-1
  Makes Cross Product Matrix : Reshape  OutputDimensionality=Customize  OutputDimensions=[3,3]
  Vector Concatenate : Concatenate  NumInputs=9
  Psi_x : Outport
  wires:
  Demux1/1 -> [v1]
  [v1] -> Gain1/1
  Gain3/1 -> Vector Concatenate/4
  Constant2/1 -> Vector Concatenate/5
  [v1] -> Vector Concatenate/6
  [v2] -> Vector Concatenate/7
  Constant1/1 -> Vector Concatenate/1
  [v3] -> Vector Concatenate/2
  Demux1/2 -> [v2]
  Vector Concatenate/1 -> Makes Cross Product Matrix/1
  Gain1/1 -> Vector Concatenate/8
  Gain/1 -> Vector Concatenate/3
  Psi_vec/1 -> Demux1/1
  Makes Cross Product Matrix/1 -> Psi_x/1
  Demux1/3 -> [v3]
  [v2] -> Gain/1
  [v3] -> Gain3/1
  Constant3/1 -> Vector Concatenate/9

== system Gyro_Outage_Unit_Test/MEKF_lib2/Time Propagation (q,P)/Psi ==
  del_t : Inport
  omega_vec : Inport  Port=2
  omega_mag : Inport  Port=3
  If : If  IfExpression=u1<1e-10
  If Action Subsystem : Subsystem  TreatAsAtomicUnit=on
  If Action Subsystem1 : Subsystem  TreatAsAtomicUnit=on
  Merge : Merge
  Psi1 : Outport
  wires:
  omega_mag/1 -> If/1, If Action Subsystem/3(omega_mag)
  del_t/1 -> If Action Subsystem/1(del_t)
  omega_vec/1 -> If Action Subsystem/2(omega_vec)
  Merge/1 -> Psi1/1
  If Action Subsystem1/1(Psi_zero) -> Merge/1
  If/1 -> If Action Subsystem1/Action
  If Action Subsystem/1(Psi) -> Merge/2
  If/2 -> If Action Subsystem/Action

== system Gyro_Outage_Unit_Test/MEKF_lib2/Time Propagation (q,P)/Subsystem ==
  del_t : Inport
  Psi_cross : Inport  Port=2
  Psi_vector : Inport  Port=3
  omega_magnitude : Inport  Port=4
  Add1 : Sum  Inputs=+-
  Constant : Constant  Value=0.5
  Cos : Trigonometry  Operator=cos
  Gain : Gain  Gain=-1
  Identity Matrix : S-Function  AncestorBlock=dspmtrx3/Identity Matrix  FunctionName=sdspeye  Parameters=Inherit,N,Ts,isCustomFloat,fxpIsSigned,dTypeID,fxpWordLength,fxpFracLength,1  SFunctionDeploymentMode=off  EnableBusSupport=off  mask(Identity Matrix){Inherit=off, N=3, Ts=1, additionalParams=off, allowOverrides=on, dataType=double, isSigned=on, wordLen=16, udDataType=sfix(16), fracBitsMode=Best precision, numFracBits=15, OutDataTypeStr=double, LastOutDataTypeStr=double}
      mask prompts: Inherit "Inherit output port attributes from input port"; N "Matrix size:"; Ts "Sample time:"; additionalParams "------- Show additional parameters --------"; allowOverrides "Allow overrides by DSP Fixed-Point Attributes blocks"; dataType "Output data type:"; isSigned "Signed"; wordLen "Word length:"; udDataType "User-defined data type (e.g. sfix(16), float('single')):"; fracBitsMode "Set fraction length in output to:"; numFracBits "Fraction length:"; OutDataTypeStr "Output data type:"; LastOutDataTypeStr "Last output data type:"
      mask help: Output an identity matrix. If the matrix size entered is a scalar, then the output will be a square (symmetric) identity matrix with the number of rows and columns both equal to the specified value. If the matrix size entered is a two-element vector [M N], then the output will be an asymmetric matrix with the number of rows equal to M, the number of columns equal to N, ones down the diagonal, and zeros elsewhere. This matches the syntax of the MATLAB function eye(N) and eye(M,N), respectively.
      mask init: same as Gyro_Outage_Unit_Test/MEKF_lib1/Time Propagation (q,P)/Subsystem/Identity Matrix
      mask Help: eval('blocksethelp');
      mask Callback Inherit: dspblkeye
      mask TypeOptions dataType: double | single | int8 | uint8 | int16 | uint16 | int32 | uint32 | boolean | Fixed-point | User-defined | Inherit via back propagation
      mask TypeOptions fracBitsMode: Best precision | User-defined
      mask Display:
      | if Inherit
      |     disp('eye( )');
      | else
      |     disp(['eye(' , num2str(get_param(gcbh, 'N')), ')']);
      | end
  Matrix Concatenate : Concatenate  Mode=Multidimensional array  ConcatenateDimension=2
  Matrix Concatenate1 : Concatenate  Mode=Multidimensional array  ConcatenateDimension=2
  Matrix Concatenate2 : Concatenate  Mode=Multidimensional array
  Matrix Multiply2 : Product
  Multiply : Product  Inputs=3
  Transpose2 : Math  Operator=transpose  SaturateOnIntegerOverflow=on
  OMEGA : Outport
  wires:
  Gain/1 -> Transpose2/1
  Constant/1 -> Multiply/2
  omega_magnitude/1 -> Multiply/3
  del_t/1 -> Multiply/1
  Identity Matrix/1 -> Matrix Multiply2/2
  Psi_cross/1 -> Add1/2
  Transpose2/1 -> Matrix Concatenate/2
  Cos/1 -> Matrix Multiply2/1, Matrix Concatenate/1
  Psi_vector/1 -> Matrix Concatenate1/1, Gain/1
  Matrix Concatenate/1 -> Matrix Concatenate2/1
  Matrix Concatenate1/1 -> Matrix Concatenate2/2
  Add1/1 -> Matrix Concatenate1/2
  Matrix Multiply2/1 -> Add1/1
  Multiply/1 -> Cos/1
  Matrix Concatenate2/1 -> OMEGA/1

== system Gyro_Outage_Unit_Test/MEKF_lib2/Triad/Bypass Triad ==
  quat_old : Inport
  Action Port : ActionPort  ActionType=else
  quat_new : Outport
  wires:
  quat_old/1 -> quat_new/1

== system Gyro_Outage_Unit_Test/MEKF_lib2/Triad/Triad_alg ==
  sun_body : Inport
  mag_body : Inport  Port=2
  "mag_inertial " : Inport  Port=3
  sun_inertial : Inport  Port=4
  Action Port : ActionPort  ActionType=then
  Cross Product{4..7} (4 alike) : vrlib/Utilities/Cross Product
      settings: SourceProductBaseCode=VR
  Determinant of 3x3 Matrix : sharedutil/Determinant of 3x3 Matrix  aMode=aMode
      settings: SourceProductName=Aerospace Blockset  SourceProductBaseCode=AE
  Direction Cosine Matrix to Quaternions2 : sharedtransform/Direction Cosine Matrix  to Quaternions  aMode=0  action=None  tolerance=eps(2)
      settings: SourceProductName=Aerospace Blockset  SourceProductBaseCode=AE
  Math Function1 : Math  Operator=transpose  SaturateOnIntegerOverflow=on
  Matrix Concatenate2 : Concatenate  NumInputs=3  Mode=Multidimensional array  ConcatenateDimension=2
  Matrix Concatenate3 : Concatenate  NumInputs=3  Mode=Multidimensional array  ConcatenateDimension=2
  Matrix Multiply1 : Product  Multiplication=Matrix(*)
  Multiply : Product
  Normalization6 : dspmathops/Normalization  NormType=2-norm  Bias=1e-10  NormOver=Each column  Dimension=1  roundingMode=Floor  overflowMode=off  accumDataTypeStr=Inherit: Same as product output  accumLastDataTypeStr=Inherit: Same as product output  outputDataTypeStr=Inherit: Same as product output  outputMin=[]  outputMax=[]  outputLastDataTypeStr=Inherit: Same as product output
      settings: SourceProductName=DSP System Toolbox
  Normalization7 : dspmathops/Normalization  NormType=2-norm  Bias=1e-10  NormOver=Each column  Dimension=1  roundingMode=Floor  overflowMode=off  accumDataTypeStr=Inherit: Same as product output  accumLastDataTypeStr=Inherit: Same as product output  outputDataTypeStr=Inherit: Same as product output  outputMin=[]  outputMax=[]  outputLastDataTypeStr=Inherit: Same as product output
      settings: SourceProductName=DSP System Toolbox
  Scope : Scope
  Selector : Selector  InputPortWidth=4  IndexOptions=Index vector (dialog)  Indices=[1]  OutputSizes=1
  Sign : Signum
  quat_out 2 : Outport
  wires:
  Multiply/1 -> quat_out 2/1
  Selector/1 -> Sign/1
  Sign/1 -> Multiply/1
  Direction Cosine Matrix to Quaternions2/1 -> Selector/1, Multiply/2
  [dcm_Inert] -> Matrix Multiply1/2
  [dcm_body] -> Matrix Multiply1/1
  Math Function1/1 -> [dcm_Inert]
  Matrix Concatenate2/1 -> [dcm_body]
  Matrix Multiply1/1 -> Determinant of 3x3 Matrix/1, Direction Cosine Matrix to Quaternions2/1
  Matrix Concatenate3/1 -> Math Function1/1
  "mag_inertial "/1 -> Cross Product6/2
  Cross Product6/1 -> Normalization7/1  "S x M"
  Normalization7/1 -> Cross Product7/2, Matrix Concatenate3/2  "M"
  Cross Product7/1 -> Matrix Concatenate3/3  "S x M"
  sun_inertial/1 -> Cross Product7/1, Matrix Concatenate3/1, Cross Product6/1
  Cross Product5/1 -> Matrix Concatenate2/3  "S x M"
  Normalization6/1 -> Cross Product5/2, Matrix Concatenate2/2  "M"
  Cross Product4/1 -> Normalization6/1  "S x M"
  mag_body/1 -> Cross Product4/2
  sun_body/1 -> Cross Product4/1, Cross Product5/1, Matrix Concatenate2/1
  Determinant of 3x3 Matrix/1 -> Scope/1
